simulink model "ret1"  (R2013a)
settings: Solver=ode23tb  StartTime=0.0  StopTime=4  RelTol=1e-3
values from neighbouring files (symbols this model uses):
  alfa = 90    [dcmsi.m]
  J = 1.1e-4    (= 0.00011)    [dcmsi.m]
  kt = 0.038    [dcmsi.m]
  La = 6.67e-4    (= 0.000667)    [dcmsi.m]
  Ra = 1.6    [dcmsi.m]
  V_source = 24*sqrt(2)    [dcmsi.m]
libraries: powerlib x7
settings Model: Creator=dello  LastModifiedBy=dello
settings DataIOCC: SignalLoggingSaveFormat=ModelDataLogs  SignalLoggingName=results
settings OptimizationCC: BlockReduction=off

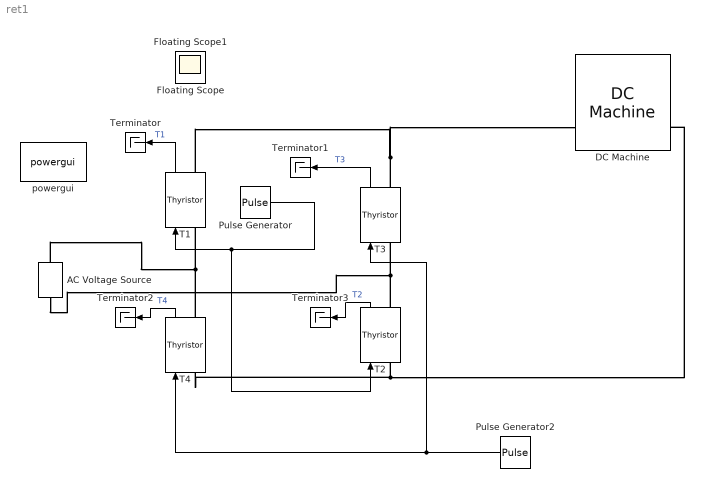
== system ret1 ==
  AC Voltage Source : powerlib/Electrical Sources/AC Voltage Source  Amplitude=V_source  Phase=0  Frequency=60  SampleTime=0  Measurements=Voltage
  DC Machine : powerlib/Machines/DC Machine  PresetModel=No  MechanicalLoad=Torque TL  FieldType=Permanent magnet  ShowDetailedParameters=on  RLa="[ Ra  La]"  RLf="[ 240  120]"  Laf=1.8  MachineConstant=Torque constant (N.m/A)  Ke=1.8  Kt=kt  J=J  Bm=B  Tf=0  w0=0  Ifinit=1  TsPowergui=0  TsBlock=-1
  Pulse Generator : DiscretePulseGenerator  PulseType=Time based  Period=1/60  PulseWidth=50  PhaseDelay=alfa/360/60
  Pulse Generator2 : DiscretePulseGenerator  PulseType=Time based  Period=1/60  PulseWidth=50  PhaseDelay=(alfa + 180)/360/60
  T{1..4} (4 alike) : powerlib/Power Electronics/Thyristor  Ron=0.001  Lon=0  Vf=0.8  IC=0  Rs=500  Cs=250e-9  Measurements=on
  Terminator{,1..3} (4 alike) : Terminator
  powergui : powerlib/powergui  Priority=1  SimulationMode=Continuous  SolverType=Tustin  SampleTime=50e-6  frequency=60  SPID=off  DisableSnubberDevices=off  DisableRonSwitches=off  DisableVfSwitches=off  SwTol=0  Interpol=off  DisplayEquations=off  frequencyindice=60  Pbase=100e6  ErrMax=1e-4  Iterations=50  UnitsV=V  UnitsW=W  FunctionMessages=off  echomessages=off  HookPort=off  EnableUseOfTLC=off  x0status=blocks  RestoreLinks=warning  ResistiveCurrentMeasurement=off  Frange=[0:2:500]  Ylog=off  Xlog=on  ShowGrid=off  save=off  variable=ZData  ZoomFFT=off  StartTime=0.0  cycles=1  DisplayStyle=1  fundamental=60  FreqAxis=off  MaxFrequency=1000  frequencyindicesteady=1  RmsSteady=1  display=off  Ts=0  methode=off
  Floating Scope : Scope  NumInputPorts=8
      settings: Floating=on  TimeRange=0.03333333333333333  YMin=-5~-5~-5~-5~-5~-5~-5~-5  YMax=5~5~5~5~5~5~5~5  SaveName=diodes
  Floating Scope1 : Scope
      settings: Floating=on  TimeRange=0.03333333333333333  SaveName=simdata
  wires:
  T1/1 -> Terminator/1  "T1"
  T3/1 -> Terminator1/1  "T3"
  T2/1 -> Terminator3/1  "T2"
  T4/1 -> Terminator2/1  "T4"
  Pulse Generator/1 -> T2/1, T1/1
  Pulse Generator2/1 -> T3/1, T4/1
  connections:
  AC Voltage Source/RConn1 -- T4/RConn1 -- T1/LConn1
  AC Voltage Source/LConn1 -- T2/RConn1 -- T3/LConn1
  T3/RConn1 -- DC Machine/LConn1 -- T1/RConn1
  T4/LConn1 -- DC Machine/RConn1 -- T2/LConn1
